simulink model "Closed Loop Control of Separately Excited DC Motor"  (R2018a)
settings: Solver=ode23tb  StartTime=0.0  StopTime=10  RelTol=1e-4
libraries: simulink x1
Description:
  | Copyright 2008-2016 The MathWorks, Inc.
settings Model: ExtModeTrigMode=oneshot  ExtModeArmWhenConnect=off  ExtModeAutoUpdateStatusClock=off  Creator=MathWorks  LastModifiedBy=User
settings SolverCC: ZeroCrossAlgorithm=Adaptive
settings DataIOCC: Decimation=5  FinalStateName=x50  InitialState=x50  MaxDataPoints=500000  SaveFormat=Array  SignalLoggingSaveFormat=ModelDataLogs  SaveOutput=off  TimeSaveName=t  SignalLoggingName=sigsOut
settings OptimizationCC: BlockReduction=off  BooleanDataType=off  ExpressionDepthLimit=2147483647  InitFltsAndDblsToZero=on  EfficientMapNaN2IntZero=off  LifeSpan=inf
settings DebuggingCC: UnderspecifiedInitializationDetection=Classic  MergeDetectMultiDrivingBlocksExec=none  CheckExecutionContextPreStartOutputMsg=on  CheckExecutionContextRuntimeOutputMsg=on  SignalResolutionControl=TryResolveAllWithWarning  MultiTaskDSMMsg=warning  MultiTaskCondExecSysMsg=none  SigSpecEnsureSampleTimeMsg=none  IntegerOverflowMsg=none  FcnCallInpInsideContextMsg=warning  StateNameClashWarn=warning  SFUnexpectedBacktrackingDiag=warning  SFNoUnconditionalDefaultTransitionDiag=warning  SFExecutionAtInitializationDiag=none  IntegerSaturationMsg=none
settings HardwareCC: ProdBitPerPointer=32  ProdBitPerSizeT=32  ProdBitPerPtrDiffT=32  ProdLargestAtomicFloat=None  ProdIntDivRoundTo=Undefined  ProdEndianess=Unspecified  ProdWordSize=32  ProdHWDeviceType=32-bit Generic  TargetUnknown=on
settings ModelReferenceCC: PropagateSignalLabelsOutOfModel=off
settings CodeAppCC: StateflowObjectComments=on
settings GRTTargetCC: TargetLangStandard=C89/C90 (ANSI)  GeneratePreprocessorConditionals=Disable all  CombineOutputUpdateFcns=off  GRTInterface=on
settings ConfigComp: CovMetricSettings=dw  CovHtmlReporting=on  CovSaveCumulativeToWorkspaceVar=on  CovSaveSingleToWorkspaceVar=on  CovExternalEMLEnable=off  CovSFcnEnable=off
settings SimscapeCC: SimscapeNormalizeSystem=off

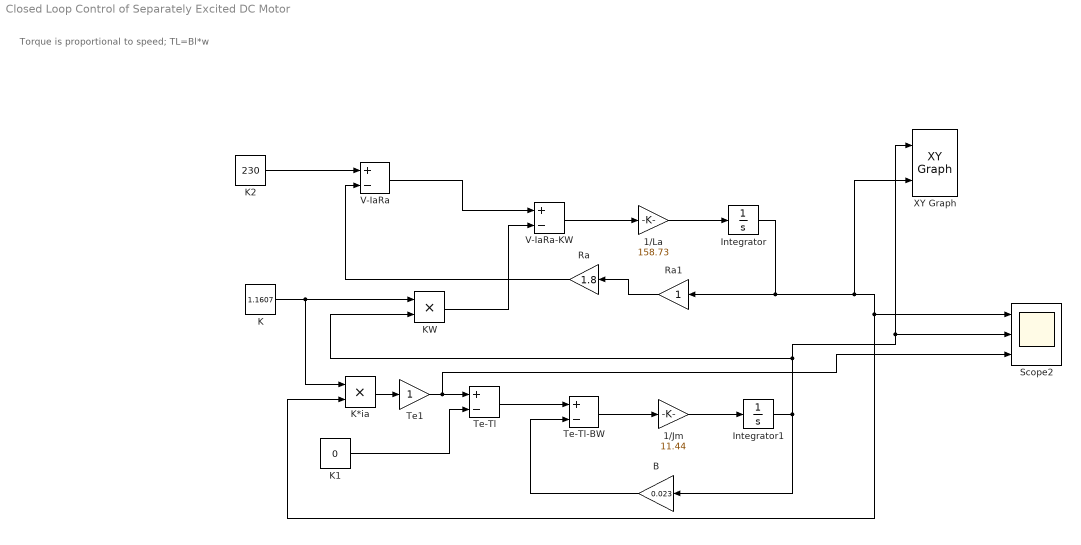
== system Closed Loop Control of Separately Excited DC Motor ==
  note: Torque is proportional to speed; TL=Bl*w
  1/Jm : Gain  Gain=11.44
  1/La : Gain  Gain=158.73
  B : Gain  Gain=0.023
  Integrator : Integrator
  Integrator1 : Integrator
  K : Constant  Value=1.1607
  K*ia : Product
  K1 : Constant  Value=0
  K2 : Constant  Value=230
  KW : Product
  Ra : Gain  Gain=1.8
  Ra1 : Gain
  Scope2 : Scope  NumInputPorts=3
  Te-Tl : Sum  Inputs=+-
  Te-Tl-BW : Sum  Inputs=+-
  Te1 : Gain
  V-IaRa : Sum  Inputs=+-
  V-IaRa-KW : Sum  Inputs=+-
  XY Graph : simulink/Sinks/XY Graph  xmin=0  xmax=40  ymin=0  ymax=140  st=-1
  wires:
  Ra/1 -> V-IaRa/2
  V-IaRa/1 -> V-IaRa-KW/1
  V-IaRa-KW/1 -> 1/La/1
  1/La/1 -> Integrator/1
  K*ia/1 -> Te1/1
  K/1 -> K*ia/1, KW/1
  Te-Tl/1 -> Te-Tl-BW/1
  Te-Tl-BW/1 -> 1/Jm/1
  1/Jm/1 -> Integrator1/1
  B/1 -> Te-Tl-BW/2
  Integrator1/1 -> B/1, KW/2, XY Graph/1, Scope2/2
  KW/1 -> V-IaRa-KW/2
  Te1/1 -> Scope2/3, Te-Tl/1
  Integrator/1 -> Ra1/1, XY Graph/2, K*ia/2, Scope2/1
  K1/1 -> Te-Tl/2
  Ra1/1 -> Ra/1
  K2/1 -> V-IaRa/1
